simulink library "Feeder4_lib"  (Simulink 8.1)
settings: Solver=ode45  StartTime=0.0  StopTime=10.0  RelTol=1e-3
values from neighbouring files (symbols this model uses):
  F4 = xlsread('F4_relay_nrel.xlsx')    [relay_settings_init.m]
  Ts = 100E-6    (= 0.0001)    [BANSHEE_init.m]
undefined symbols (not defined in the file or in its folder): CBID, DER_REL, Left, type, V
libraries: breaker_lib x9, Load_lib x7, cables_lib x3, relay_modbus_lib x3, rtio_generic_modbus x3, NREL_Diesel_Genset_lib x2, BESS_lib x2, rtlab x2, ssn_lib x2, powerlib x1, transformer_lib x1
settings Model: Creator=re25624  LastModifiedBy=pkoralew

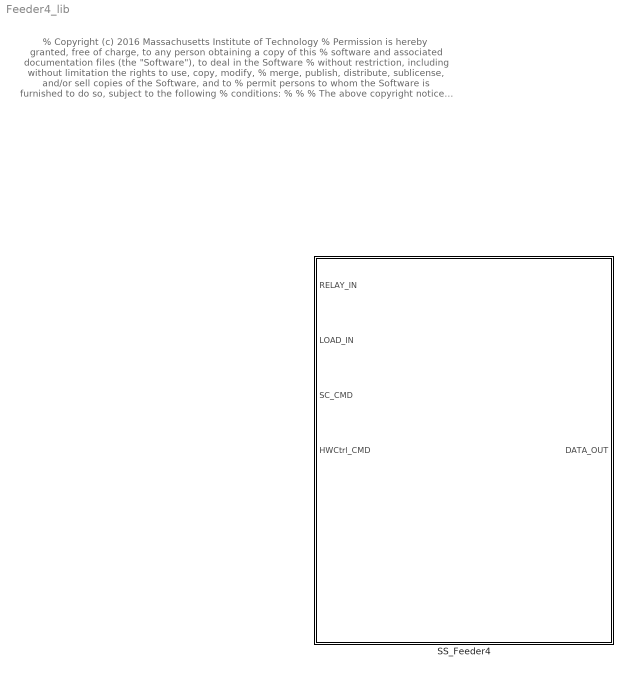
== system Feeder4_lib ==
  note: % Copyright (c) 2016 Massachusetts Institute of Technology
      | % Permission is hereby granted, free of charge, to any person obtaining a copy of this
      | % software and associated documentation files (the "Software"), to deal in the Software
      | % without restriction, including without limitation the rights to use, copy, modify,
      | % merge, publish, distribute, sublicense, and/or sell copies of the Software, and to
      | % permit persons to whom the Software is furnished to do so, subject to the following
      | % conditions:
      | %
      | %
      | % The above copyright notice and this permission notice shall be included in
      | % all copies or substantial portions of the Software.
      | %
      | % THE SOFTWARE IS PROVIDED "AS IS", WITHOUT WARRANTY OF ANY KIND, EXPRESS OR IMPLIED,
      | % INCLUDING BUT NOT LIMITED TO THE WARRANTIES OF MERCHANTABILITY, FITNESS FOR A
      | % PARTICULAR PURPOSE AND NONINFRINGEMENT. IN NO EVENT SHALL THE AUTHORS OR COPYRIGHT
      | % HOLDERS BE LIABLE FOR ANY CLAIM, DAMAGES OR OTHER LIABILITY, WHETHER IN AN ACTION
      | % OF CONTRACT, TORT OR OTHERWISE, ARISING FROM, OUT OF OR IN CONNECTION WITH THE
      | % SOFTWARE OR THE USE OR OTHER DEALINGS IN THE SOFTWARE.
      | %
      | %
      | %%
  SS_Feeder4 : Subsystem

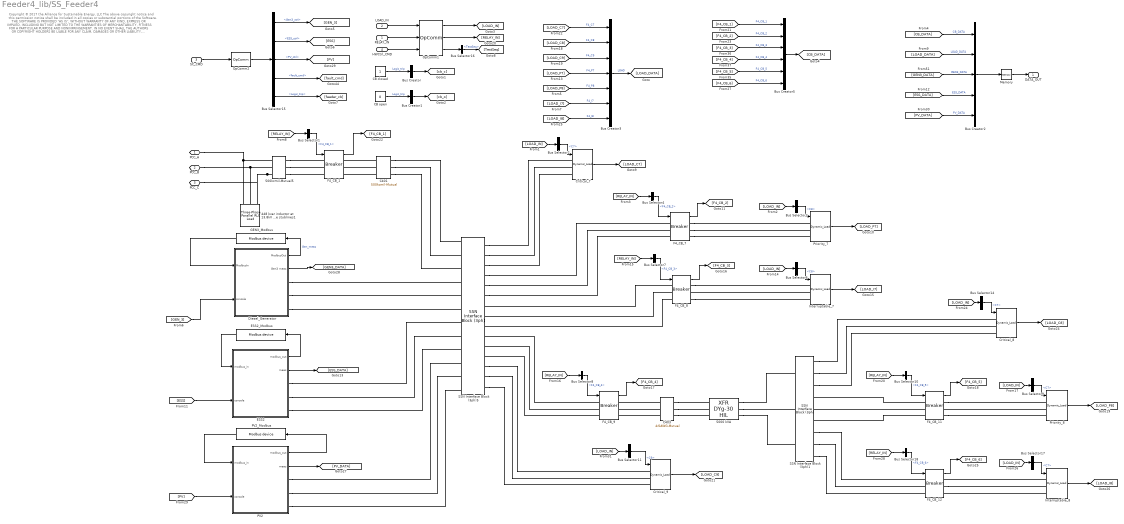
== system Feeder4_lib/SS_Feeder4 ==
  note: Copyright © 2017 the Alliance for Sustainable Energy, LLC
      |
      | The above copyright notice and this permission notice shall be included in all copies or substantial portions of the Software.
      |
      | THE SOFTWARE IS PROVIDED "AS IS", WITHOUT WARRANTY OF ANY KIND, EXPRESS OR IMPLIED, INCLUDING
      | BUT NOT LIMITED TO THE WARRANTIES OF MERCHANTABILITY, FITNESS FOR A PARTICULAR PURPOSE AND
      | NONINFRINGEMENT. IN NO EVENT SHALL THE AUTHORS OR COPYRIGHT HOLDERS BE LIABLE FOR ANY CLAIM,
      |  DAMAGES OR OTHER LIABILITY, WHETHER IN AN ACTION OF CONTRACT, TORT OR OTHERWISE, ARISING FROM,
      | OUT OF OR IN CONNECTION WITH THE SOFTWARE OR THE USE OR OTHER DEALINGS IN THE SOFTWARE
  RELAY_IN : Inport
  LOAD_IN : Inport  Port=2
  SC_CMD : Inport  Port=3
  HWCtrl_CMD : Inport  Port=4
  448 kvar inductor at 13.8kV  to cancel kvar produced by the stublines1 : powerlib/Elements/Three-Phase Parallel RLC Load  LConnTagsString=A|B|C  Configuration=Y (grounded)  NominalVoltage=13800  NominalFrequency=60  ActivePower=0  InductivePower=448e3  CapacitivePower=0  Measurements=None  LoadType=constant Z
  5000 kVA : transformer_lib/XFR DYg-30 HIL  Rating=50  Vp=480  Vs=208  Z=5.75  XR=4.7
  500kcmil-Mutual5 : cables_lib/500kcmil-Mutual  length=1000  par_sets=1  ratio=3
  Bus Creator : BusCreator  Inputs=1
  Bus Creator1 : BusCreator  Inputs=1
  Bus Creator2 : BusCreator  Inputs=5
  Bus Creator3 : BusCreator  Inputs=7
  Bus Creator5 : BusCreator  Inputs=6
  Bus Selector1 : BusSelector  OutputSignals=F4_CB_1
  Bus Selector10 : BusSelector  OutputSignals=F4_CB_5
  Bus Selector11 : BusSelector  OutputSignals=C9
  Bus Selector{2,9,14,17} (4 alike) : BusSelector  OutputSignals=C7
  Bus Selector15 : BusSelector  OutputSignals=Gen3_ctrl,ESS_ctrl,PV_ctrl,fault_cmd,GridStatusCtrl.Grid_F3.Logic_trip
  Bus Selector16 : BusSelector  OutputSignals=TestSeq
  Bus Selector18 : BusSelector  OutputSignals=F4_CB_6
  Bus Selector3 : BusSelector  OutputSignals=C8
  Bus Selector4 : BusSelector  OutputSignals=F4_CB_2
  Bus Selector6 : BusSelector  OutputSignals=C8
  Bus Selector7 : BusSelector  OutputSignals=F4_CB_3
  Bus Selector8 : BusSelector  OutputSignals=F4_CB_4
  C401 : cables_lib/500kcmil-Mutual  length=2000  par_sets=1  ratio=3
  C403 : cables_lib/4//0AWG-Mutual  length=2000  par_sets=1  ratio=3
  CB closed : Constant
  CB open : Constant  Value=0
  Critical_7 : Load_lib/Dynamic_Load  V=480  kVA=25  PF=0.9  Ts=Ts
  Critical_8 : Load_lib/Dynamic_Load  V=208  kVA=20  PF=0.9  Ts=Ts
  Critical_9 : Load_lib/Dynamic_Load  V=480  kVA=3  PF=0.9  Ts=Ts
  Diesel_Generator : Subsystem
  ESS2 : Subsystem
  ESS2_Modbus : rtio_generic_modbus/Modbus device  conf_name=ESS2_modbus.opal  conf_name_mask=ESS2_modbus.xls  sample_time=Ts
  F4_CB_{1,7..9,11..12} (6 alike) : breaker_lib/Breaker  Ts=Ts  mech_delay=cb_mech_delay
  GEN3_Modbus : rtio_generic_modbus/Modbus device  conf_name=GEN3_modbus.opal  conf_name_mask=GEN3_modbus.xls  sample_time=Ts
  Interruptable_7 : Load_lib/Dynamic_Load  V=480  kVA=30  PF=0.9  Ts=Ts
  Interruptable_8 : Load_lib/Dynamic_Load  V=208  kVA=20  PF=0.9  Ts=Ts
  Memory : Memory
  OpComm1 : rtlab/OpComm  nbport=3  groupe_acq=1  subsys_rate=0  st=0  Synchronization=on  Interpolation=on  Threshold=1.0  Missed_Data=off  Sim_Time=off  Samples=off  dynSigOut=off  from_console=0  warning_done=off  writeOpCommFile=off  Offset=off
  OpComm2 : rtlab/OpComm  nbport=1  groupe_acq=1  subsys_rate=0  st=0  Synchronization=on  Interpolation=on  Threshold=1.0  Missed_Data=off  Sim_Time=off  Samples=off  dynSigOut=off  from_console=1  warning_done=off  writeOpCommFile=off  Offset=off
  PV2 : Subsystem
  PV2_Modbus : rtio_generic_modbus/Modbus device  conf_name=PV2_modbus.opal  conf_name_mask=PV2_modbus.xls  sample_time=Ts
  Priority_7 : Load_lib/Dynamic_Load  V=480  kVA=10  PF=0.9  Ts=Ts
  Priority_8 : Load_lib/Dynamic_Load  V=208  kVA=10  PF=0.9  Ts=Ts
  SSN Interface Block (3ph)1 : ssn_lib/SSN Interface Block (3ph)  nb_phase=3  nb_port=4  p1_type=V-type(Left)  p2_type=V-type (Right)  p3_type=V-type (Right)  p4_type=V-type (Right)  p5_type=V-type (Right)  p6_type=V-type (Right)  p7_type=V-type (Right)  p8_type=V-type(Left)  p9_type=V-type(Left)  p10_type=V-type(Left)  p11_type=V-type(Left)  p12_type=V-type(Left)  p13_type=V-type(Left)  p14_type=V-type(Left)  p15_type=V-type(Left)  p16_type=V-type(Left)  I_port_shunt_resistance=1e9
  SSN Interface Block (3ph)5 : ssn_lib/SSN Interface Block (3ph)  nb_phase=3  nb_port=9  p1_type=V-type(Left)  p2_type=V-type (Right)  p3_type=V-type (Right)  p4_type=V-type (Right)  p5_type=V-type (Right)  p6_type=V-type (Right)  p7_type=V-type(Left)  p8_type=V-type(Left)  p9_type=V-type(Left)  p10_type=V-type(Left)  p11_type=V-type(Left)  p12_type=V-type(Left)  p13_type=V-type(Left)  p14_type=V-type(Left)  p15_type=V-type(Left)  p16_type=V-type(Left)  I_port_shunt_resistance=1e9
  PCC_A : PMIOPort  Port=1  Side=Left
  PCC_B : PMIOPort  Port=2  Side=Left
  PCC_C : PMIOPort  Port=3  Side=Left
  DATA_OUT : Outport
  wires:
  [LOAD_I8] -> Bus Creator3/7  "F4_I8"
  [LOAD_P8] -> Bus Creator3/5  "F4_P8"
  [LOAD_P7] -> Bus Creator3/4  "F4_P7"
  [LOAD_I7] -> Bus Creator3/6  "F4_I7"
  Diesel_Generator/2(Gen3 meas) -> [GEN3_DATA]
  Diesel_Generator/1(ModbusOut) -> GEN3_Modbus/1  "Gen_meas"
  GEN3_Modbus/1 -> Diesel_Generator/1(ModbusIn)
  ESS2_Modbus/1 -> ESS2/1(modbus_in)
  ESS2/1(modbus_out) -> ESS2_Modbus/1
  ESS2/2(meas) -> [ESS_DATA]
  PV2/2(meas) -> [PV_DATA]
  PV2/1(modbus_out) -> PV2_Modbus/1
  [PV] -> PV2/2(console)
  PV2_Modbus/1 -> PV2/1(modbus_in)
  Bus Selector15/3 -> [PV]  "<PV_ctrl>"
  [PV_DATA] -> Bus Creator2/5  "PV_DATA"
  F4_CB_12/1 -> [F4_CB_6]
  Bus Selector18/1 -> F4_CB_12/1  "<F4_CB_6>"
  [RELAY_IN] -> Bus Selector18/1
  [LOAD_IN] -> Bus Selector17/1
  Bus Selector17/1 -> Interruptable_8/1  "<C7>"
  Interruptable_8/1 -> [LOAD_I8]
  [LOAD_IN] -> Bus Selector14/1
  Bus Selector14/1 -> Critical_8/1  "<C7>"
  Critical_8/1 -> [LOAD_C8]
  F4_CB_11/1 -> [F4_CB_5]
  Bus Selector10/1 -> F4_CB_11/1  "<F4_CB_5>"
  [RELAY_IN] -> Bus Selector10/1
  [LOAD_IN] -> Bus Selector9/1
  Bus Selector9/1 -> Priority_8/1  "<C7>"
  Priority_8/1 -> [LOAD_P8]
  F4_CB_9/1 -> [F4_CB_4]
  Bus Selector8/1 -> F4_CB_9/1  "<F4_CB_4>"
  [RELAY_IN] -> Bus Selector8/1
  F4_CB_8/1 -> [F4_CB_3]
  Bus Selector7/1 -> F4_CB_8/1  "<F4_CB_3>"
  [RELAY_IN] -> Bus Selector7/1
  [LOAD_IN] -> Bus Selector6/1
  Bus Selector6/1 -> Interruptable_7/1  "<C8>"
  Interruptable_7/1 -> [LOAD_I7]
  [ESS] -> ESS2/2(console)
  [ESS_DATA] -> Bus Creator2/4  "ESS_DATA"
  Bus Selector1/1 -> F4_CB_1/1  "<F4_CB_1>"
  [RELAY_IN] -> Bus Selector1/1
  Bus Selector15/2 -> [ESS]  "<ESS_ctrl>"
  [GEN_3] -> Diesel_Generator/2(console)
  F4_CB_7/1 -> [F4_CB_2]
  Bus Selector4/1 -> F4_CB_7/1  "<F4_CB_2>"
  [RELAY_IN] -> Bus Selector4/1
  [LOAD_IN] -> Bus Selector3/1
  Bus Selector3/1 -> Priority_7/1  "<C8>"
  Priority_7/1 -> [LOAD_P7]
  [LOAD_IN] -> Bus Selector2/1
  Bus Selector2/1 -> Critical_7/1  "<C7>"
  Critical_7/1 -> [LOAD_C7]
  [LOAD_IN] -> Bus Selector11/1
  Bus Selector11/1 -> Critical_9/1  "<C9>"
  Critical_9/1 -> [LOAD_C9]
  CB closed/1 -> Bus Creator/1  "Logic_trip"
  Bus Creator/1 -> [cb_c]
  Bus Creator1/1 -> [cb_o]
  CB open/1 -> Bus Creator1/1  "Logic_trip"
  LOAD_IN/1 -> OpComm1/1
  OpComm1/1 -> [LOAD_IN]
  [LOAD_C8] -> Bus Creator3/2  "F4_C8"
  [LOAD_C7] -> Bus Creator3/1  "F4_C7"
  [LOAD_C9] -> Bus Creator3/3  "F4_C9"
  Bus Creator3/1 -> [LOAD_DATA]  "LOAD"
  [F4_CB_1] -> Bus Creator5/1  "F4_CB_1"
  [F4_CB_5] -> Bus Creator5/5  "F4_CB_5"
  [F4_CB_6] -> Bus Creator5/6  "F4_CB_6"
  [F4_CB_3] -> Bus Creator5/3  "F4_CB_3"
  [F4_CB_2] -> Bus Creator5/2  "F4_CB_2"
  [F4_CB_4] -> Bus Creator5/4  "F4_CB_4"
  Bus Creator5/1 -> [CB_DATA]
  RELAY_IN/1 -> OpComm1/2
  OpComm1/2 -> [RELAY_IN]
  F4_CB_1/1 -> [F4_CB_1]
  SC_CMD/1 -> OpComm2/1
  Memory/1 -> DATA_OUT/1
  OpComm2/1 -> Bus Selector15/1
  Bus Selector15/4 -> [fault_cmd]  "<fault_cmd>"
  HWCtrl_CMD/1 -> OpComm1/3
  OpComm1/3 -> Bus Selector16/1
  Bus Creator2/1 -> Memory/1
  [CB_DATA] -> Bus Creator2/1  "CB_DATA"
  [LOAD_DATA] -> Bus Creator2/2  "LOAD_DATA"
  [GEN3_DATA] -> Bus Creator2/3  "GEN3_DATA"
  Bus Selector15/1 -> [GEN_3]  "<Gen3_ctrl>"
  Bus Selector15/5 -> [feeder_cb]  "<Logic_trip>"
  Bus Selector16/1 -> [TestSeq]  "<TestSeq>"
  connections:
  SSN Interface Block (3ph)5/RConn13 -- Critical_9/LConn1
  SSN Interface Block (3ph)5/RConn14 -- Critical_9/LConn2
  SSN Interface Block (3ph)5/RConn15 -- Critical_9/LConn3
  PV2/RConn3 -- SSN Interface Block (3ph)5/LConn12
  PV2/RConn2 -- SSN Interface Block (3ph)5/LConn11
  PV2/RConn1 -- SSN Interface Block (3ph)5/LConn10
  ESS2/RConn2 -- SSN Interface Block (3ph)5/LConn8
  ESS2/RConn1 -- SSN Interface Block (3ph)5/LConn7
  ESS2/RConn3 -- SSN Interface Block (3ph)5/LConn9
  Diesel_Generator/RConn3 -- SSN Interface Block (3ph)5/LConn6
  Diesel_Generator/RConn2 -- SSN Interface Block (3ph)5/LConn5
  Diesel_Generator/RConn1 -- SSN Interface Block (3ph)5/LConn4
  SSN Interface Block (3ph)1/RConn7 -- F4_CB_12/LConn1
  SSN Interface Block (3ph)1/RConn8 -- F4_CB_12/LConn2
  SSN Interface Block (3ph)1/RConn9 -- F4_CB_12/LConn3
  F4_CB_11/LConn1 -- SSN Interface Block (3ph)1/RConn4
  F4_CB_11/LConn2 -- SSN Interface Block (3ph)1/RConn5
  F4_CB_11/LConn3 -- SSN Interface Block (3ph)1/RConn6
  SSN Interface Block (3ph)1/RConn1 -- Critical_8/LConn1
  SSN Interface Block (3ph)1/RConn2 -- Critical_8/LConn2
  SSN Interface Block (3ph)1/RConn3 -- Critical_8/LConn3
  F4_CB_12/RConn2 -- Interruptable_8/LConn2
  Interruptable_8/LConn3 -- F4_CB_12/RConn3
  Interruptable_8/LConn1 -- F4_CB_12/RConn1
  F4_CB_11/RConn3 -- Priority_8/LConn3
  F4_CB_11/RConn1 -- Priority_8/LConn1
  Priority_8/LConn2 -- F4_CB_11/RConn2
  5000 kVA/RConn1 -- SSN Interface Block (3ph)1/LConn1
  5000 kVA/RConn3 -- SSN Interface Block (3ph)1/LConn3
  5000 kVA/RConn2 -- SSN Interface Block (3ph)1/LConn2
  C403/RConn3 -- 5000 kVA/LConn3
  C403/RConn1 -- 5000 kVA/LConn1
  C403/RConn2 -- 5000 kVA/LConn2
  F4_CB_9/LConn2 -- SSN Interface Block (3ph)5/RConn11
  F4_CB_9/LConn1 -- SSN Interface Block (3ph)5/RConn10
  F4_CB_9/LConn3 -- SSN Interface Block (3ph)5/RConn12
  C403/LConn2 -- F4_CB_9/RConn2
  C403/LConn3 -- F4_CB_9/RConn3
  C403/LConn1 -- F4_CB_9/RConn1
  Interruptable_7/LConn2 -- F4_CB_8/RConn2
  F4_CB_8/RConn3 -- Interruptable_7/LConn3
  F4_CB_8/RConn1 -- Interruptable_7/LConn1
  F4_CB_8/LConn3 -- SSN Interface Block (3ph)5/RConn9
  F4_CB_8/LConn2 -- SSN Interface Block (3ph)5/RConn8
  F4_CB_8/LConn1 -- SSN Interface Block (3ph)5/RConn7
  SSN Interface Block (3ph)5/RConn2 -- Critical_7/LConn2
  SSN Interface Block (3ph)5/RConn3 -- Critical_7/LConn3
  SSN Interface Block (3ph)5/RConn1 -- Critical_7/LConn1
  SSN Interface Block (3ph)5/RConn4 -- F4_CB_7/LConn1
  SSN Interface Block (3ph)5/RConn5 -- F4_CB_7/LConn2
  SSN Interface Block (3ph)5/RConn6 -- F4_CB_7/LConn3
  F4_CB_7/RConn1 -- Priority_7/LConn1
  F4_CB_7/RConn3 -- Priority_7/LConn3
  F4_CB_7/RConn2 -- Priority_7/LConn2
  C401/LConn3 -- F4_CB_1/RConn3
  C401/LConn1 -- F4_CB_1/RConn1
  C401/LConn2 -- F4_CB_1/RConn2
  500kcmil-Mutual5/RConn1 -- F4_CB_1/LConn1
  500kcmil-Mutual5/RConn2 -- F4_CB_1/LConn2
  500kcmil-Mutual5/RConn3 -- F4_CB_1/LConn3
  C401/RConn1 -- SSN Interface Block (3ph)5/LConn1
  C401/RConn2 -- SSN Interface Block (3ph)5/LConn2
  C401/RConn3 -- SSN Interface Block (3ph)5/LConn3
  PCC_A/RConn1 -- 500kcmil-Mutual5/LConn1 -- 448 kvar inductor at 13.8kV  to cancel kvar produced by the stublines1/LConn1
  PCC_B/RConn1 -- 448 kvar inductor at 13.8kV  to cancel kvar produced by the stublines1/LConn2 -- 500kcmil-Mutual5/LConn2
  500kcmil-Mutual5/LConn3 -- 448 kvar inductor at 13.8kV  to cancel kvar produced by the stublines1/LConn3 -- PCC_C/RConn1

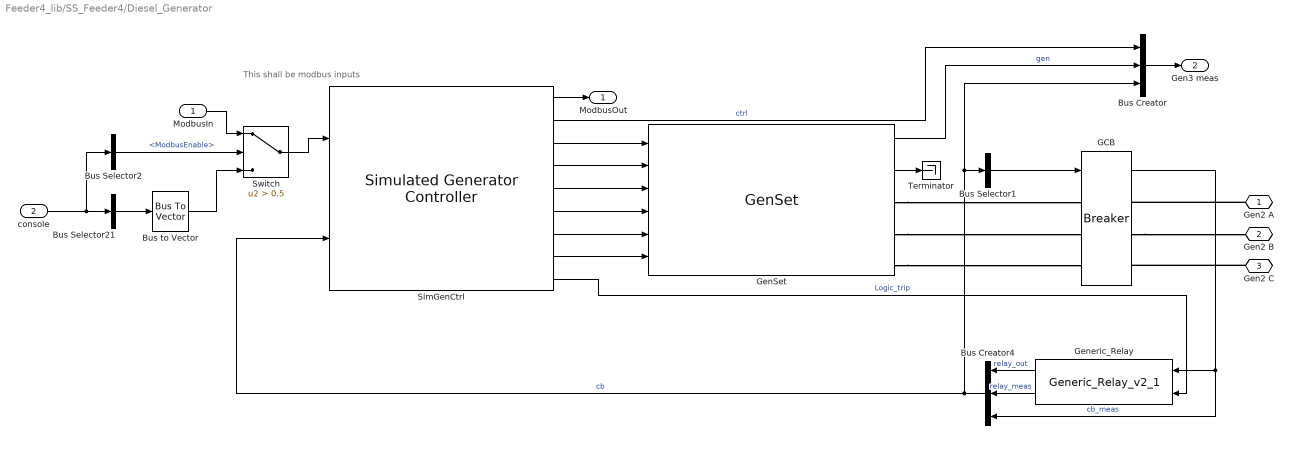
== system Feeder4_lib/SS_Feeder4/Diesel_Generator ==
  note: This shall be modbus inputs
  ModbusIn : Inport
  console : Inport  Port=2
  Bus Creator : BusCreator  Inputs=3
  Bus Creator4 : BusCreator  Inputs=3
  Bus Selector1 : BusSelector  OutputSignals=relay_out  OutputAsBus=on
  Bus Selector2 : BusSelector  OutputSignals=ModbusEnable
  Bus Selector21 : BusSelector  OutputSignals=ModbusFromSC.Ctrl,ModbusFromSC.PCmd,ModbusFromSC.QCmd,ModbusFromSC.VoltCmd,ModbusFromSC.FreqCmd,ModbusFromSC.signal6,ModbusFromSC.signal7,ModbusFromSC.signal8  OutputAsBus=on
  Bus to Vector : BusToVector
  GCB : breaker_lib/Breaker  Ts=Ts  mech_delay=cb_mech_delay
  GenSet : NREL_Diesel_Genset_lib/GenSet  GenSel=80kVA diesel generator
  Generic_Relay : relay_modbus_lib/Generic_Relay_v2_1  Ts=Ts  relay_settings=[DER_REL(CBID.GEN3,:)]
  SimGenCtrl : NREL_Diesel_Genset_lib/Simulated Generator Controller  GenSel=80kVA diesel generator
  Switch : Switch  Criteria=u2 > Threshold  Threshold=0.5
  Terminator : Terminator
  Gen2 A : PMIOPort  Port=1  Side=Right
  Gen2 B : PMIOPort  Port=2  Side=Right
  Gen2 C : PMIOPort  Port=3  Side=Right
  ModbusOut : Outport
  Gen3 meas : Outport  Port=2
  wires:
  SimGenCtrl/9 -> Generic_Relay/2  "Logic_trip"
  SimGenCtrl/1 -> ModbusOut/1
  SimGenCtrl/8 -> GenSet/6
  SimGenCtrl/7 -> GenSet/5
  SimGenCtrl/3 -> GenSet/1
  SimGenCtrl/4 -> GenSet/2
  SimGenCtrl/5 -> GenSet/3
  SimGenCtrl/6 -> GenSet/4
  GenSet/1 -> Bus Creator/2  "gen"
  Bus Creator4/1 -> Bus Creator/3, Bus Selector1/1, SimGenCtrl/2  "cb"
  console/1 -> Bus Selector21/1, Bus Selector2/1
  Bus Selector2/1 -> Switch/2  "<ModbusEnable>"
  ModbusIn/1 -> Switch/1
  Bus Selector21/1 -> Bus to Vector/1
  Bus to Vector/1 -> Switch/3
  Switch/1 -> SimGenCtrl/1
  GCB/1 -> Generic_Relay/1, Bus Creator4/3  "cb_meas"
  Generic_Relay/1 -> Bus Creator4/1  "relay_out"
  Generic_Relay/2 -> Bus Creator4/2  "relay_meas"
  Bus Creator/1 -> Gen3 meas/1
  SimGenCtrl/2 -> Bus Creator/1  "ctrl"
  Bus Selector1/1 -> GCB/1
  GenSet/2 -> Terminator/1
  connections:
  Gen2 A/RConn1 -- GCB/RConn1
  GCB/RConn2 -- Gen2 B/RConn1
  Gen2 C/RConn1 -- GCB/RConn3
  GenSet/RConn1 -- GCB/LConn1
  GenSet/RConn2 -- GCB/LConn2
  GenSet/RConn3 -- GCB/LConn3

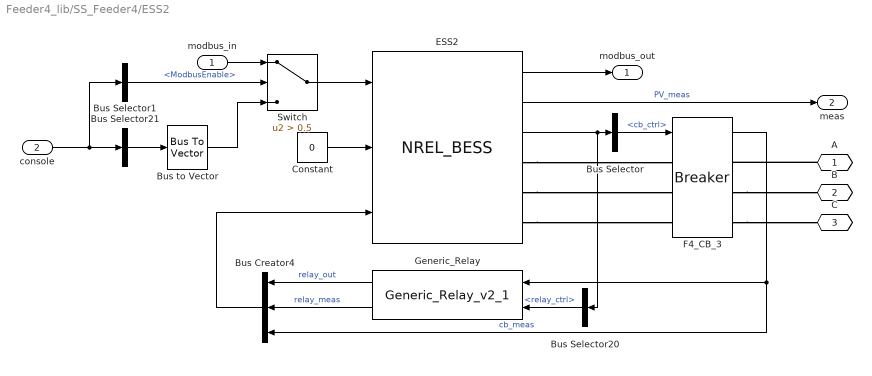
== system Feeder4_lib/SS_Feeder4/ESS2 ==
  modbus_in : Inport
  console : Inport  Port=2
  Bus Creator4 : BusCreator  Inputs=3
  Bus Selector : BusSelector  OutputSignals=cb_ctrl
  Bus Selector1 : BusSelector  OutputSignals=ModbusEnable
  Bus Selector20 : BusSelector  OutputSignals=relay_ctrl
  Bus Selector21 : BusSelector  OutputSignals=ModbusFromSC.Ctrl,ModbusFromSC.PCmd,ModbusFromSC.QCmd,ModbusFromSC.VoltCmd,ModbusFromSC.FreqCmd,ModbusFromSC.signal6,ModbusFromSC.signal7,ModbusFromSC.signal8  OutputAsBus=on
  Bus to Vector : BusToVector
  Constant : Constant  Value=0
  ESS2 : BESS_lib/NREL_BESS  InvType=ESS Inverter  Sn=250  Vn=480  b_Vdc_nom=1000  b_kWh=1  b_esr=0.1  r_I_max=3  Tc=Ts
  F4_CB_3 : breaker_lib/Breaker  Ts=Ts  mech_delay=cb_mech_delay
  Generic_Relay : relay_modbus_lib/Generic_Relay_v2_1  Ts=Ts  relay_settings=[F4(3,:)]
  Switch : Switch  Criteria=u2 > Threshold  Threshold=0.5
  A : PMIOPort  Port=1  Side=Right
  B : PMIOPort  Port=2  Side=Right
  C : PMIOPort  Port=3  Side=Right
  modbus_out : Outport
  meas : Outport  Port=2
  wires:
  Constant/1 -> ESS2/2
  Bus to Vector/1 -> Switch/3
  ESS2/3 -> Bus Selector/1, Bus Selector20/1
  F4_CB_3/1 -> Bus Creator4/3, Generic_Relay/1  "cb_meas"
  Switch/1 -> ESS2/1
  Bus Selector21/1 -> Bus to Vector/1
  modbus_in/1 -> Switch/1
  ESS2/1 -> modbus_out/1
  Bus Selector1/1 -> Switch/2  "<ModbusEnable>"
  console/1 -> Bus Selector21/1, Bus Selector1/1
  Bus Selector20/1 -> Generic_Relay/2  "<relay_ctrl>"
  Bus Selector/1 -> F4_CB_3/1  "<cb_ctrl>"
  Generic_Relay/1 -> Bus Creator4/1  "relay_out"
  ESS2/2 -> meas/1  "PV_meas"
  Generic_Relay/2 -> Bus Creator4/2  "relay_meas"
  Bus Creator4/1 -> ESS2/3
  connections:
  F4_CB_3/RConn3 -- C/RConn1
  A/RConn1 -- F4_CB_3/RConn1
  ESS2/RConn1 -- F4_CB_3/LConn1
  ESS2/RConn3 -- F4_CB_3/LConn3
  ESS2/RConn2 -- F4_CB_3/LConn2
  F4_CB_3/RConn2 -- B/RConn1

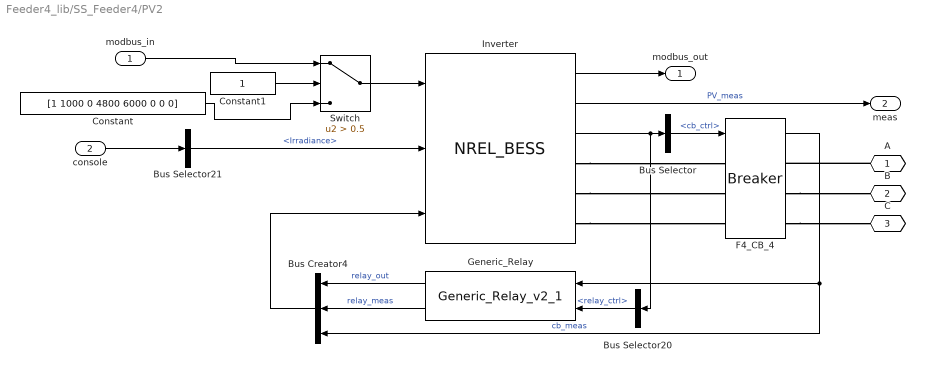
== system Feeder4_lib/SS_Feeder4/PV2 ==
  modbus_in : Inport
  console : Inport  Port=2
  Bus Creator4 : BusCreator  Inputs=3
  Bus Selector : BusSelector  OutputSignals=cb_ctrl
  Bus Selector20 : BusSelector  OutputSignals=relay_ctrl
  Bus Selector21 : BusSelector  OutputSignals=Irradiance
  Constant : Constant  Value=[1 1000 0 4800 6000 0 0 0]
  Constant1 : Constant
  F4_CB_4 : breaker_lib/Breaker  Ts=Ts  mech_delay=cb_mech_delay
  Generic_Relay : relay_modbus_lib/Generic_Relay_v2_1  Ts=Ts  relay_settings=[F4(4,:)]
  Inverter : BESS_lib/NREL_BESS  InvType=PV Inverter  Sn=100  Vn=480  b_Vdc_nom=1000  b_kWh=1  b_esr=0.1  r_I_max=1.2  Tc=Ts
  Switch : Switch  Criteria=u2 > Threshold  Threshold=0.5
  A : PMIOPort  Port=1  Side=Right
  B : PMIOPort  Port=2  Side=Right
  C : PMIOPort  Port=3  Side=Right
  modbus_out : Outport
  meas : Outport  Port=2
  wires:
  Bus Selector21/1 -> Inverter/2  "<Irradiance>"
  Bus Creator4/1 -> Inverter/3
  Generic_Relay/2 -> Bus Creator4/2  "relay_meas"
  Inverter/2 -> meas/1  "PV_meas"
  Generic_Relay/1 -> Bus Creator4/1  "relay_out"
  Bus Selector/1 -> F4_CB_4/1  "<cb_ctrl>"
  Bus Selector20/1 -> Generic_Relay/2  "<relay_ctrl>"
  console/1 -> Bus Selector21/1
  Constant1/1 -> Switch/2
  Inverter/1 -> modbus_out/1
  modbus_in/1 -> Switch/1
  Constant/1 -> Switch/3
  Switch/1 -> Inverter/1
  F4_CB_4/1 -> Generic_Relay/1, Bus Creator4/3  "cb_meas"
  Inverter/3 -> Bus Selector/1, Bus Selector20/1
  connections:
  F4_CB_4/RConn2 -- B/RConn1
  Inverter/RConn2 -- F4_CB_4/LConn2
  Inverter/RConn3 -- F4_CB_4/LConn3
  Inverter/RConn1 -- F4_CB_4/LConn1
  A/RConn1 -- F4_CB_4/RConn1
  F4_CB_4/RConn3 -- C/RConn1
